simulink model "helicopter_control_xplane_9"  (R2016a)
settings: Solver=VariableStepAuto  StartTime=0.0  StopTime=inf  RelTol=1e-3
libraries: dspindex x18, dspnetwork x4, etargetslib x2
settings Model: Creator=iwin  LastModifiedBy=iwin

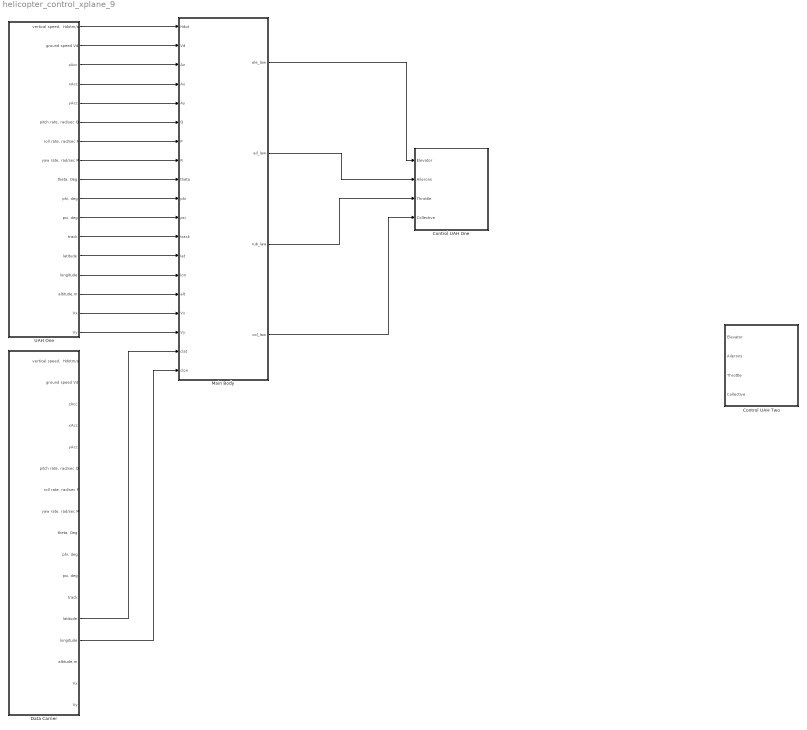
== system helicopter_control_xplane_9 ==
  Control UAH One : Subsystem  Description=|  mask(Send Commands to X-Plane 9){remoteURL='192.168.137.5', remotePort=49000}
      | Done by: Mohamed Abdelkader
      | Contact for updates: mohamedashraf123@gmail.com
      mask prompts: remoteURL "Remote X-Plane Address ('127.0.0.1')"; remotePort "Remote X-Plane Port (49000)"
      mask help:
      | Sends Control Surfaces Commands to Xplane 9
      | Throttle in [0,1]
      | Elevator, Ailerons, rudder, nosewheel in [-1,1]
      mask TypeOptions remoteURL: UDP Send/remoteURL
  Control UAH Two : Subsystem  Description=|  mask(Send Commands to X-Plane 9){remoteURL='192.168.137.6', remotePort=49000}
      | Done by: Mohamed Abdelkader
      | Contact for updates: mohamedashraf123@gmail.com
      mask prompts: remoteURL "Remote X-Plane Address ('127.0.0.1')"; remotePort "Remote X-Plane Port (49000)"
      mask help:
      | Sends Control Surfaces Commands to Xplane 9
      | Throttle in [0,1]
      | Elevator, Ailerons, rudder, nosewheel in [-1,1]
      mask TypeOptions remoteURL: UDP Send/remoteURL
  Data Carrier : Subsystem  Description=|  TreatAsAtomicUnit=on  mask(Get Data from Xplane10){remoteURL='192.168.137.6', localPort=49005, sampletime=0.02}
      | Done by: Mohamed Abdelkader
      | Contact for updates: mohamedashraf123@gmail.com
      mask prompts: remoteURL "Remote IP address ('0.0.0.0' to accept all):(default='127.0.0.1')"; localPort "Local IP port: that Xplane10 sends to (default=49005)"; sampletime "Sampling time (seconds), how frequenlty to capture data from Xplane. Don't set to low as it might not be able to capture the smaples from Xplane. Default is 0.02 assuming the UDP rate in Xplane is set to 50 sample per second"
      mask help:
      | Get Data from X-Plane10
      | * make sure you configure the right port
      | and the right IP address
      mask TypeOptions remoteURL: UDP Receive1/remoteURL
      mask TypeOptions localPort: UDP Receive1/localPort
      mask TypeOptions sampletime: UDP Receive1/sampletime
  Main Body : Subsystem  mask(Controller for Helicoper){PSICMD=0, VYCMD=0, VXCMD=0, HCMD=12}
      mask prompts: PSICMD "Give the yaw angle"; VYCMD "Give the latitude velocity"; VXCMD "Give the longitude velocity"; HCMD "Give the height"
      mask help: Control the Helicopter in X-Plane 9
  UAH One : Subsystem  Description=|  TreatAsAtomicUnit=on  mask(Get Data from Xplane10){remoteURL='192.168.137.5', localPort=49005, sampletime=0.02}
      | Done by: Mohamed Abdelkader
      | Contact for updates: mohamedashraf123@gmail.com
      mask prompts: remoteURL "Remote IP address ('0.0.0.0' to accept all):(default='127.0.0.1')"; localPort "Local IP port: that Xplane10 sends to (default=49005)"; sampletime "Sampling time (seconds), how frequenlty to capture data from Xplane. Don't set to low as it might not be able to capture the smaples from Xplane. Default is 0.02 assuming the UDP rate in Xplane is set to 50 sample per second"
      mask help:
      | Get Data from X-Plane10
      | * make sure you configure the right port
      | and the right IP address
      mask TypeOptions remoteURL: UDP Receive1/remoteURL
      mask TypeOptions localPort: UDP Receive1/localPort
      mask TypeOptions sampletime: UDP Receive1/sampletime
  wires:
  Main Body/1(ele_law) -> Control UAH One/1(Elevator)
  Main Body/2(ail_law) -> Control UAH One/2(Ailerons)
  Main Body/3(rub_law) -> Control UAH One/3(Throttle)
  Main Body/4(col_law) -> Control UAH One/4(Collective)
  UAH One/1("vertical speed,  Hdotm/s") -> Main Body/1(Hdot)
  UAH One/2(ground speed Vd) -> Main Body/2(Vd)
  UAH One/3(zAcc) -> Main Body/3(Az)
  UAH One/4(xAcc) -> Main Body/4(Ax)
  UAH One/5(yAcc) -> Main Body/5(Ay)
  UAH One/6("pitch rate, rad/sec Q") -> Main Body/6(Q)
  UAH One/7(" roll rate, rad/sec P") -> Main Body/7(P)
  UAH One/8("yaw rate, rad/sec R") -> Main Body/8(R)
  UAH One/9("theta, Deg") -> Main Body/9(theta)
  UAH One/10("phi, deg") -> Main Body/10(phi)
  UAH One/11("psi, deg") -> Main Body/11(psi)
  UAH One/12(track) -> Main Body/12(track)
  UAH One/13(latitude) -> Main Body/13(lat)
  UAH One/14(longitude) -> Main Body/14(lon)
  UAH One/15(altitude,m) -> Main Body/15(alt)
  UAH One/16(Vx) -> Main Body/16(Vx)
  UAH One/17(Vy) -> Main Body/17(Vy)
  Data Carrier/13(latitude) -> Main Body/18(clat)
  Data Carrier/14(longitude) -> Main Body/19(clon)

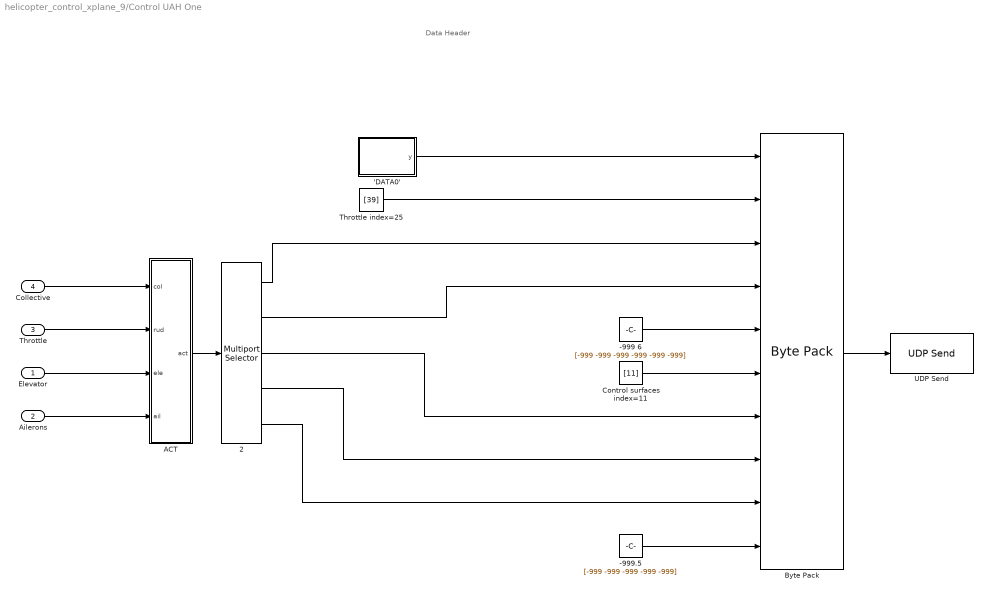
== system helicopter_control_xplane_9/Control UAH One ==
  note: Data Header
  Elevator : Inport
  Ailerons : Inport  Port=2
  Throttle : Inport  Port=3
  Collective : Inport  Port=4
  'DATA0' : MATLAB Function  TreatAsAtomicUnit=on
  -999 6 : Constant  Value=[-999 -999 -999 -999 -999 -999]  OutDataTypeStr=int32  SampleTime=-1
  -999.5 : Constant  Value=[-999 -999 -999 -999 -999]  OutDataTypeStr=int32  SampleTime=-1
  2 : dspindex/Multiport Selector  rowsOrCols=Columns  idxCellArray={1 2 3 4 5}  idxErrMode=Clip Index
  ACT : MATLAB Function  TreatAsAtomicUnit=on
  Byte Pack : etargetslib/Byte Pack  datatypes={'uint8','uint32','single','single','int32','uint32','single','single','single','int32'}  byteAlign=1
  Control surfaces index=11 : Constant  Value=[11]  OutDataTypeStr=uint32  SampleTime=-1
  Throttle index=25 : Constant  Value=[39]  OutDataTypeStr=uint32  SampleTime=-1
  UDP Send : dspnetwork/UDP Send  remoteURL=remoteURL  remotePort=49000  localURL='0.0.0.0'  localPortSource=Automatically determine  localPort=-1  sampletime=-1  separateLengthPort=0
  wires:
  Byte Pack/1 -> UDP Send/1
  Throttle index=25/1 -> Byte Pack/2
  'DATA0'/1(y) -> Byte Pack/1
  -999 6/1 -> Byte Pack/5
  Control surfaces index=11/1 -> Byte Pack/6
  -999.5/1 -> Byte Pack/10
  2/1 -> Byte Pack/3
  2/2 -> Byte Pack/4
  ACT/1(act) -> 2/1
  Collective/1 -> ACT/1(col)
  Elevator/1 -> ACT/3(ele)
  Throttle/1 -> ACT/2(rud)
  Ailerons/1 -> ACT/4(ail)
  2/3 -> Byte Pack/7
  2/4 -> Byte Pack/8
  2/5 -> Byte Pack/9

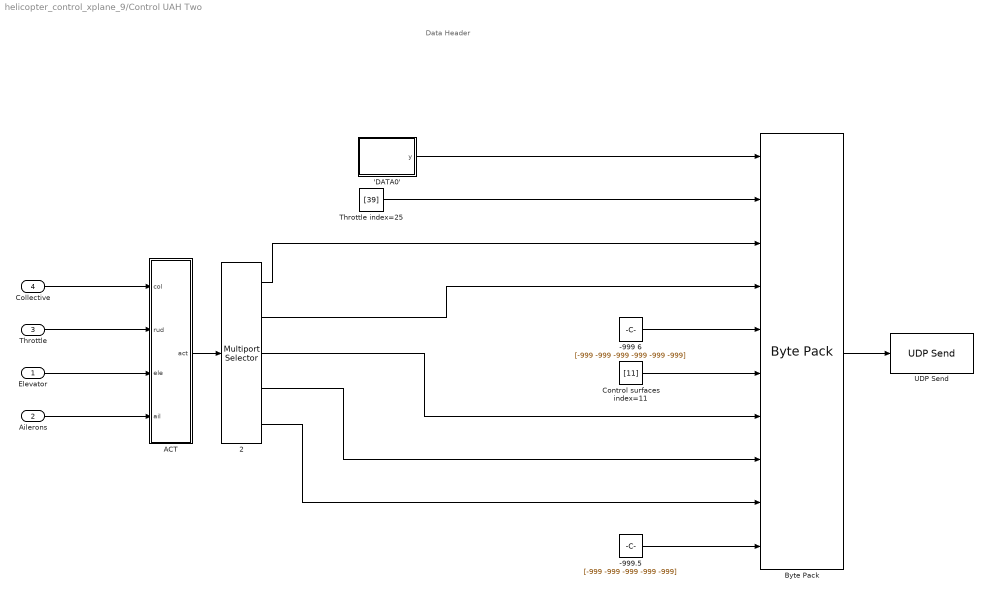
== system helicopter_control_xplane_9/Control UAH Two ==
  note: Data Header
  Elevator : Inport
  Ailerons : Inport  Port=2
  Throttle : Inport  Port=3
  Collective : Inport  Port=4
  'DATA0' : MATLAB Function  TreatAsAtomicUnit=on
  -999 6 : Constant  Value=[-999 -999 -999 -999 -999 -999]  OutDataTypeStr=int32  SampleTime=-1
  -999.5 : Constant  Value=[-999 -999 -999 -999 -999]  OutDataTypeStr=int32  SampleTime=-1
  2 : dspindex/Multiport Selector  rowsOrCols=Columns  idxCellArray={1 2 3 4 5}  idxErrMode=Clip Index
  ACT : MATLAB Function  TreatAsAtomicUnit=on
  Byte Pack : etargetslib/Byte Pack  datatypes={'uint8','uint32','single','single','int32','uint32','single','single','single','int32'}  byteAlign=1
  Control surfaces index=11 : Constant  Value=[11]  OutDataTypeStr=uint32  SampleTime=-1
  Throttle index=25 : Constant  Value=[39]  OutDataTypeStr=uint32  SampleTime=-1
  UDP Send : dspnetwork/UDP Send  remoteURL=remoteURL  remotePort=49000  localURL='0.0.0.0'  localPortSource=Automatically determine  localPort=-1  sampletime=-1  separateLengthPort=0
  wires:
  2/5 -> Byte Pack/9
  2/4 -> Byte Pack/8
  2/3 -> Byte Pack/7
  Ailerons/1 -> ACT/4(ail)
  Throttle/1 -> ACT/2(rud)
  Elevator/1 -> ACT/3(ele)
  Collective/1 -> ACT/1(col)
  ACT/1(act) -> 2/1
  2/2 -> Byte Pack/4
  2/1 -> Byte Pack/3
  -999.5/1 -> Byte Pack/10
  Control surfaces index=11/1 -> Byte Pack/6
  -999 6/1 -> Byte Pack/5
  'DATA0'/1(y) -> Byte Pack/1
  Throttle index=25/1 -> Byte Pack/2
  Byte Pack/1 -> UDP Send/1

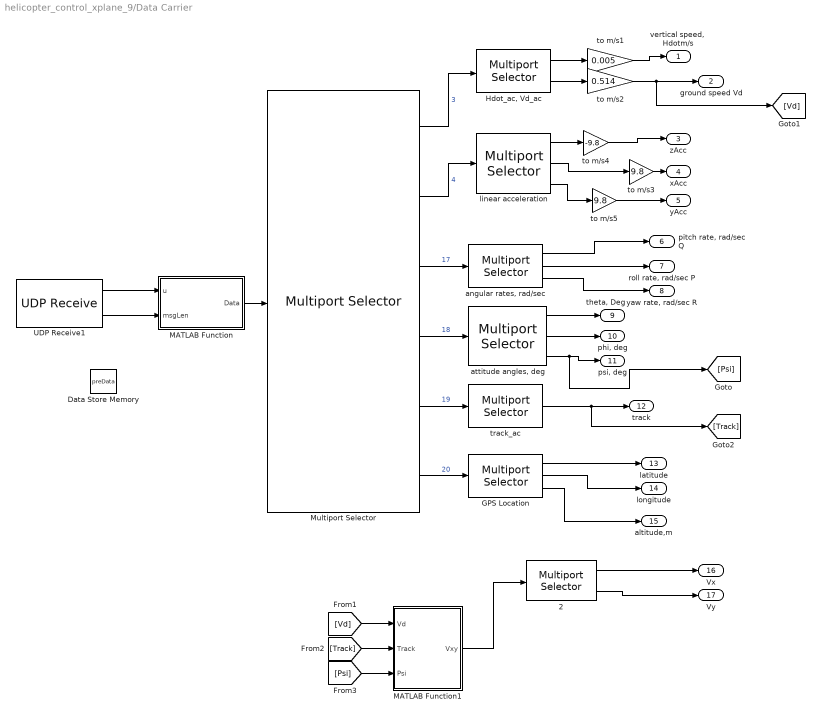
== system helicopter_control_xplane_9/Data Carrier ==
  2 : dspindex/Multiport Selector  rowsOrCols=Columns  idxCellArray={1 2}  idxErrMode=Clip Index
  Data Store Memory : DataStoreMemory  DataStoreName=preData  InitialValue=zeros(140, 8)  ShowAdditionalParam=off  OutDataTypeStr=single
  GPS Location : dspindex/Multiport Selector  rowsOrCols=Columns  idxCellArray={1,2,3}  idxErrMode=Clip Index
  "Hdot_ac, Vd_ac" : dspindex/Multiport Selector  rowsOrCols=Columns  idxCellArray={5, 7}  idxErrMode=Clip Index
  MATLAB Function : MATLAB Function  TreatAsAtomicUnit=on
  MATLAB Function1 : MATLAB Function  TreatAsAtomicUnit=on
  Multiport Selector : dspindex/Multiport Selector  rowsOrCols=Rows  idxCellArray={3,4,17,18,19,20}  idxErrMode=Clip Index
  UDP Receive1 : dspnetwork/UDP Receive  localURL='0.0.0.0'  localPort=localPort  remoteURL=remoteURL  remotePort=-1  recvBufferSize=8192  dims=365*20  signalDatatype=uint8  isVarSize=off  showBlockingTime=off  blockingTime=0  sampletime=sampletime
  "angular rates, rad/sec" : dspindex/Multiport Selector  rowsOrCols=Columns  idxCellArray={1,2,3}  idxErrMode=Clip Index
  "attitude angles, deg" : dspindex/Multiport Selector  rowsOrCols=Columns  idxCellArray={1, 2, 3}  idxErrMode=Clip Index
  linear acceleration : dspindex/Multiport Selector  rowsOrCols=Columns  idxCellArray={3, 4, 5}  idxErrMode=Clip Index
  to m/s1 : Gain  Gain=0.005  OutDataTypeStr=double
  to m/s2 : Gain  Gain=0.514
  to m/s3 : Gain  Gain=9.8
  to m/s4 : Gain  Gain=-9.8
  to m/s5 : Gain  Gain=9.8
  track_ac : dspindex/Multiport Selector  rowsOrCols=Columns  idxCellArray={3}  idxErrMode=Clip Index
  "vertical speed,  Hdotm/s" : Outport  OutDataTypeStr=double
  ground speed Vd : Outport  Port=2
  zAcc : Outport  Port=3
  xAcc : Outport  Port=4
  yAcc : Outport  Port=5
  "pitch rate, rad/sec Q" : Outport  Port=6
  " roll rate, rad/sec P" : Outport  Port=7
  "yaw rate, rad/sec R" : Outport  Port=8
  "theta, Deg" : Outport  Port=9
  "phi, deg" : Outport  Port=10
  "psi, deg" : Outport  Port=11
  track : Outport  Port=12
  latitude : Outport  Port=13
  longitude : Outport  Port=14
  altitude,m : Outport  Port=15
  Vx : Outport  Port=16
  Vy : Outport  Port=17
  wires:
  2/2 -> Vy/1
  2/1 -> Vx/1
  MATLAB Function1/1(Vxy) -> 2/1
  [Vd] -> MATLAB Function1/1(Vd)
  [Track] -> MATLAB Function1/2(Track)
  [Psi] -> MATLAB Function1/3(Psi)
  track_ac/1 -> track/1, [Track]
  "attitude angles, deg"/1 -> "theta, Deg"/1
  "angular rates, rad/sec"/1 -> "pitch rate, rad/sec Q"/1
  to m/s5/1 -> yAcc/1
  linear acceleration/3 -> to m/s5/1
  linear acceleration/2 -> to m/s3/1
  to m/s4/1 -> zAcc/1
  to m/s2/1 -> ground speed Vd/1, [Vd]
  to m/s1/1 -> "vertical speed,  Hdotm/s"/1
  "Hdot_ac, Vd_ac"/2 -> to m/s2/1
  "Hdot_ac, Vd_ac"/1 -> to m/s1/1
  Multiport Selector/6 -> GPS Location/1  "20"
  Multiport Selector/5 -> track_ac/1  "19"
  Multiport Selector/4 -> "attitude angles, deg"/1  "18"
  Multiport Selector/3 -> "angular rates, rad/sec"/1  "17"
  "attitude angles, deg"/2 -> "phi, deg"/1
  "attitude angles, deg"/3 -> "psi, deg"/1, [Psi]
  UDP Receive1/2 -> MATLAB Function/2(msgLen)
  UDP Receive1/1 -> MATLAB Function/1(u)
  GPS Location/3 -> altitude,m/1
  to m/s3/1 -> xAcc/1
  "angular rates, rad/sec"/2 -> " roll rate, rad/sec P"/1
  GPS Location/1 -> latitude/1
  linear acceleration/1 -> to m/s4/1
  GPS Location/2 -> longitude/1
  Multiport Selector/1 -> "Hdot_ac, Vd_ac"/1  "3"
  MATLAB Function/1(Data) -> Multiport Selector/1
  "angular rates, rad/sec"/3 -> "yaw rate, rad/sec R"/1
  Multiport Selector/2 -> linear acceleration/1  "4"

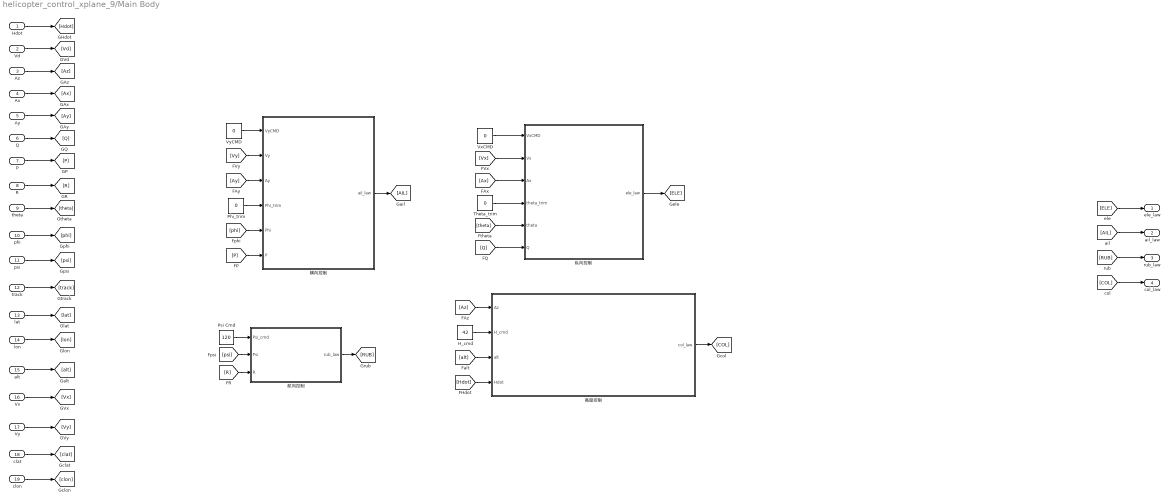
== system helicopter_control_xplane_9/Main Body ==
  Hdot : Inport
  Vd : Inport  Port=2
  Az : Inport  Port=3
  Ax : Inport  Port=4
  Ay : Inport  Port=5
  Q : Inport  Port=6
  P : Inport  Port=7
  R : Inport  Port=8
  theta : Inport  Port=9
  phi : Inport  Port=10
  psi : Inport  Port=11
  track : Inport  Port=12
  lat : Inport  Port=13
  lon : Inport  Port=14
  alt : Inport  Port=15
  Vx : Inport  Port=16
  Vy : Inport  Port=17
  clat : Inport  Port=18
  clon : Inport  Port=19
  H_cmd : Constant  Value=42  OutDataTypeStr=single
  Phi_trim : Constant  Value=0  OutDataTypeStr=single
  Psi Cmd : Constant  Value=120  OutDataTypeStr=single
  Theta_trim : Constant  Value=0  OutDataTypeStr=single
  VxCMD : Constant  Value=0  OutDataTypeStr=single
  VyCMD : Constant  Value=0  OutDataTypeStr=single
  横向控制 : Subsystem
  纵向控制 : Subsystem
  航向控制 : Subsystem
  高度控制 : Subsystem
  ele_law : Outport
  ail_law : Outport  Port=2
  rub_law : Outport  Port=3
  col_law : Outport  Port=4
  wires:
  Hdot/1 -> [Hdot]
  Vd/1 -> [Vd]
  Az/1 -> [Az]
  Ax/1 -> [Ax]
  Ay/1 -> [Ay]
  Q/1 -> [Q]
  P/1 -> [P]
  R/1 -> [R]
  theta/1 -> [theta]
  phi/1 -> [phi]
  psi/1 -> [psi]
  track/1 -> [track]
  lat/1 -> [lat]
  lon/1 -> [lon]
  alt/1 -> [alt]
  [ELE] -> ele_law/1
  [AIL] -> ail_law/1
  [RUB] -> rub_law/1
  [COL] -> col_law/1
  Vx/1 -> [Vx]
  Vy/1 -> [Vy]
  [Az] -> 高度控制/1(Az)
  H_cmd/1 -> 高度控制/2(H_cmd)
  [alt] -> 高度控制/3(alt)
  [Hdot] -> 高度控制/4(Hdot)
  高度控制/1(col_law) -> [COL]
  Psi Cmd/1 -> 航向控制/1(Psi_cmd)
  [psi] -> 航向控制/2(Psi)
  [R] -> 航向控制/3(R)
  航向控制/1(rub_law) -> [RUB]
  VyCMD/1 -> 横向控制/1(VyCMD)
  [Vy] -> 横向控制/2(Vy)
  [Ay] -> 横向控制/3(Ay)
  Phi_trim/1 -> 横向控制/4(Phi_trim)
  [phi] -> 横向控制/5(Phi)
  [P] -> 横向控制/6(P)
  横向控制/1(ail_law) -> [AIL]
  VxCMD/1 -> 纵向控制/1(VxCMD)
  [Vx] -> 纵向控制/2(Vx)
  [Ax] -> 纵向控制/3(Ax)
  Theta_trim/1 -> 纵向控制/4(theta_trim)
  [theta] -> 纵向控制/5(theta)
  [Q] -> 纵向控制/6(Q)
  纵向控制/1(ele_law) -> [ELE]
  clat/1 -> [clat]
  clon/1 -> [clon]

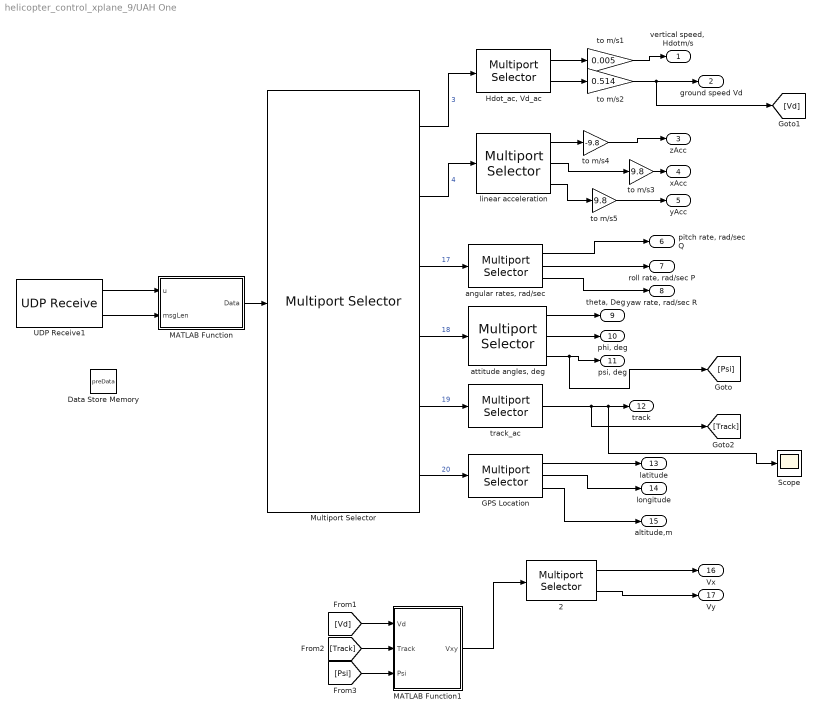
== system helicopter_control_xplane_9/UAH One ==
  2 : dspindex/Multiport Selector  rowsOrCols=Columns  idxCellArray={1 2}  idxErrMode=Clip Index
  Data Store Memory : DataStoreMemory  DataStoreName=preData  InitialValue=zeros(140, 8)  ShowAdditionalParam=off  OutDataTypeStr=single
  GPS Location : dspindex/Multiport Selector  rowsOrCols=Columns  idxCellArray={1,2,3}  idxErrMode=Clip Index
  "Hdot_ac, Vd_ac" : dspindex/Multiport Selector  rowsOrCols=Columns  idxCellArray={5, 7}  idxErrMode=Clip Index
  MATLAB Function : MATLAB Function  TreatAsAtomicUnit=on
  MATLAB Function1 : MATLAB Function  TreatAsAtomicUnit=on
  Multiport Selector : dspindex/Multiport Selector  rowsOrCols=Rows  idxCellArray={3,4,17,18,19,20}  idxErrMode=Clip Index
  Scope : Scope
  UDP Receive1 : dspnetwork/UDP Receive  localURL='0.0.0.0'  localPort=localPort  remoteURL=remoteURL  remotePort=-1  recvBufferSize=8192  dims=365*20  signalDatatype=uint8  isVarSize=off  showBlockingTime=off  blockingTime=0  sampletime=sampletime
  "angular rates, rad/sec" : dspindex/Multiport Selector  rowsOrCols=Columns  idxCellArray={1,2,3}  idxErrMode=Clip Index
  "attitude angles, deg" : dspindex/Multiport Selector  rowsOrCols=Columns  idxCellArray={1, 2, 3}  idxErrMode=Clip Index
  linear acceleration : dspindex/Multiport Selector  rowsOrCols=Columns  idxCellArray={3, 4, 5}  idxErrMode=Clip Index
  to m/s1 : Gain  Gain=0.005  OutDataTypeStr=double
  to m/s2 : Gain  Gain=0.514
  to m/s3 : Gain  Gain=9.8
  to m/s4 : Gain  Gain=-9.8
  to m/s5 : Gain  Gain=9.8
  track_ac : dspindex/Multiport Selector  rowsOrCols=Columns  idxCellArray={3}  idxErrMode=Clip Index
  "vertical speed,  Hdotm/s" : Outport  OutDataTypeStr=double
  ground speed Vd : Outport  Port=2
  zAcc : Outport  Port=3
  xAcc : Outport  Port=4
  yAcc : Outport  Port=5
  "pitch rate, rad/sec Q" : Outport  Port=6
  " roll rate, rad/sec P" : Outport  Port=7
  "yaw rate, rad/sec R" : Outport  Port=8
  "theta, Deg" : Outport  Port=9
  "phi, deg" : Outport  Port=10
  "psi, deg" : Outport  Port=11
  track : Outport  Port=12
  latitude : Outport  Port=13
  longitude : Outport  Port=14
  altitude,m : Outport  Port=15
  Vx : Outport  Port=16
  Vy : Outport  Port=17
  wires:
  Multiport Selector/2 -> linear acceleration/1  "4"
  "angular rates, rad/sec"/3 -> "yaw rate, rad/sec R"/1
  MATLAB Function/1(Data) -> Multiport Selector/1
  Multiport Selector/1 -> "Hdot_ac, Vd_ac"/1  "3"
  GPS Location/2 -> longitude/1
  linear acceleration/1 -> to m/s4/1
  GPS Location/1 -> latitude/1
  "angular rates, rad/sec"/2 -> " roll rate, rad/sec P"/1
  to m/s3/1 -> xAcc/1
  GPS Location/3 -> altitude,m/1
  UDP Receive1/1 -> MATLAB Function/1(u)
  UDP Receive1/2 -> MATLAB Function/2(msgLen)
  "attitude angles, deg"/3 -> [Psi], "psi, deg"/1
  "attitude angles, deg"/2 -> "phi, deg"/1
  Multiport Selector/3 -> "angular rates, rad/sec"/1  "17"
  Multiport Selector/4 -> "attitude angles, deg"/1  "18"
  Multiport Selector/5 -> track_ac/1  "19"
  Multiport Selector/6 -> GPS Location/1  "20"
  "Hdot_ac, Vd_ac"/1 -> to m/s1/1
  "Hdot_ac, Vd_ac"/2 -> to m/s2/1
  to m/s1/1 -> "vertical speed,  Hdotm/s"/1
  to m/s2/1 -> [Vd], ground speed Vd/1
  to m/s4/1 -> zAcc/1
  linear acceleration/2 -> to m/s3/1
  linear acceleration/3 -> to m/s5/1
  to m/s5/1 -> yAcc/1
  "angular rates, rad/sec"/1 -> "pitch rate, rad/sec Q"/1
  "attitude angles, deg"/1 -> "theta, Deg"/1
  track_ac/1 -> [Track], Scope/1, track/1
  [Psi] -> MATLAB Function1/3(Psi)
  [Track] -> MATLAB Function1/2(Track)
  [Vd] -> MATLAB Function1/1(Vd)
  MATLAB Function1/1(Vxy) -> 2/1
  2/1 -> Vx/1
  2/2 -> Vy/1

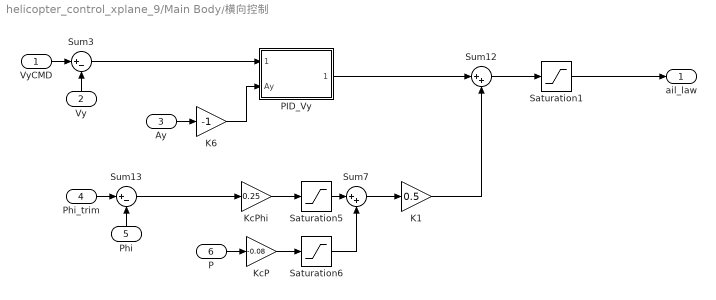
== system helicopter_control_xplane_9/Main Body/横向控制 ==
  VyCMD : Inport
  Vy : Inport  Port=2
  Ay : Inport  Port=3
  Phi_trim : Inport  Port=4
  Phi : Inport  Port=5
  P : Inport  Port=6
  K1 : Gain  Gain=0.5  OutDataTypeStr=single
  K6 : Gain  Gain=-1
  KcP : Gain  Gain=-0.08
  KcPhi : Gain  Gain=0.25  OutDataTypeStr=single
  PID_Vy : Subsystem
  Saturation1 : Saturate  UpperLimit=5.0  LowerLimit=-5.0
  Saturation5 : Saturate  UpperLimit=30  LowerLimit=-30
  Saturation6 : Saturate  UpperLimit=50  LowerLimit=-50
  Sum12 : Sum  Inputs=|++  AccumDataTypeStr=single  OutDataTypeStr=single  InputSameDT=on
  Sum13 : Sum  Inputs=|+-  OutDataTypeStr=double  InputSameDT=on
  Sum3 : Sum  Inputs=|+-  OutDataTypeStr=double  InputSameDT=on
  Sum7 : Sum  Inputs=|++  AccumDataTypeStr=single  OutDataTypeStr=double  InputSameDT=on
  ail_law : Outport
  wires:
  K6/1 -> PID_Vy/2(Ay)
  KcPhi/1 -> Saturation5/1
  Sum13/1 -> KcPhi/1
  KcP/1 -> Saturation6/1
  PID_Vy/1(AIL_FFC) -> Sum12/1
  Sum7/1 -> K1/1
  Saturation6/1 -> Sum7/2
  Saturation5/1 -> Sum7/1
  Sum3/1 -> PID_Vy/1(Vy_delta)
  Sum12/1 -> Saturation1/1
  K1/1 -> Sum12/2
  Phi/1 -> Sum13/2
  Ay/1 -> K6/1
  P/1 -> KcP/1
  Vy/1 -> Sum3/2
  Phi_trim/1 -> Sum13/1
  Saturation1/1 -> ail_law/1
  VyCMD/1 -> Sum3/1

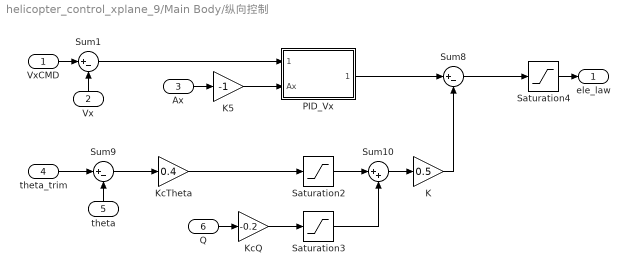
== system helicopter_control_xplane_9/Main Body/纵向控制 ==
  VxCMD : Inport
  Vx : Inport  Port=2
  Ax : Inport  Port=3
  theta_trim : Inport  Port=4
  theta : Inport  Port=5
  Q : Inport  Port=6
  K : Gain  Gain=0.5  OutDataTypeStr=single
  K5 : Gain  Gain=-1
  KcQ : Gain  Gain=-0.2
  KcTheta : Gain  Gain=0.4  OutDataTypeStr=single
  PID_Vx : Subsystem
  Saturation2 : Saturate  UpperLimit=45  LowerLimit=-45
  Saturation3 : Saturate  UpperLimit=50  LowerLimit=-50
  Saturation4 : Saturate  UpperLimit=5.0  LowerLimit=-5.0
  Sum1 : Sum  Inputs=|+-  OutDataTypeStr=double  InputSameDT=on
  Sum10 : Sum  Inputs=|++  AccumDataTypeStr=single  OutDataTypeStr=double  InputSameDT=on
  Sum8 : Sum  Inputs=|+-  AccumDataTypeStr=single  OutMin=[-1]  OutMax=[1]  OutDataTypeStr=single  InputSameDT=on
  Sum9 : Sum  Inputs=|+-  OutDataTypeStr=double  InputSameDT=on
  ele_law : Outport
  wires:
  K5/1 -> PID_Vx/2(Ax)
  Sum10/1 -> K/1
  Sum8/1 -> Saturation4/1
  PID_Vx/1(ELE_FFC) -> Sum8/1
  KcQ/1 -> Saturation3/1
  Sum1/1 -> PID_Vx/1(Vx_delta)
  Saturation2/1 -> Sum10/1
  K/1 -> Sum8/2
  KcTheta/1 -> Saturation2/1
  Saturation3/1 -> Sum10/2
  Sum9/1 -> KcTheta/1
  Vx/1 -> Sum1/2
  VxCMD/1 -> Sum1/1
  Saturation4/1 -> ele_law/1
  Ax/1 -> K5/1
  theta_trim/1 -> Sum9/1
  theta/1 -> Sum9/2
  Q/1 -> KcQ/1

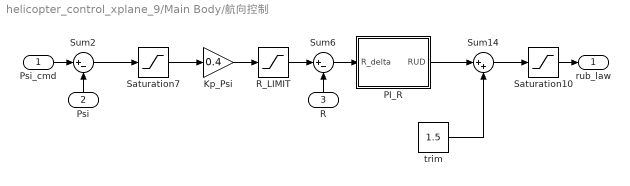
== system helicopter_control_xplane_9/Main Body/航向控制 ==
  Psi_cmd : Inport
  Psi : Inport  Port=2
  R : Inport  Port=3
  Kp_Psi : Gain  Gain=0.4  OutDataTypeStr=single
  PI_R : Subsystem
  R_LIMIT : Saturate  UpperLimit=5  LowerLimit=-5
  Saturation10 : Saturate  UpperLimit=20.0  LowerLimit=-8.0  OutDataTypeStr=single
  Saturation7 : Saturate  UpperLimit=30  LowerLimit=-30
  Sum14 : Sum  Inputs=|++  OutMin=[-1]  OutMax=[1]  OutDataTypeStr=double  InputSameDT=on
  Sum2 : Sum  Inputs=|+-  OutDataTypeStr=double  InputSameDT=on
  Sum6 : Sum  Inputs=|+-  OutDataTypeStr=double  InputSameDT=on
  trim : Constant  Value=1.5  OutDataTypeStr=single
  rub_law : Outport
  wires:
  R_LIMIT/1 -> Sum6/1
  Sum2/1 -> Saturation7/1
  trim/1 -> Sum14/2
  Kp_Psi/1 -> R_LIMIT/1
  Saturation7/1 -> Kp_Psi/1
  PI_R/1(RUD) -> Sum14/1
  Sum6/1 -> PI_R/1(R_delta)
  Sum14/1 -> Saturation10/1
  Saturation10/1 -> rub_law/1
  Psi_cmd/1 -> Sum2/1
  Psi/1 -> Sum2/2
  R/1 -> Sum6/2

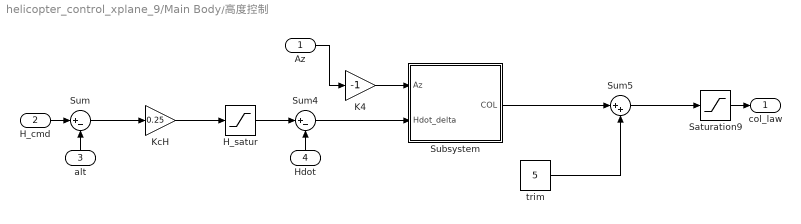
== system helicopter_control_xplane_9/Main Body/高度控制 ==
  Az : Inport
  H_cmd : Inport  Port=2
  alt : Inport  Port=3
  Hdot : Inport  Port=4
  H_satur : Saturate  UpperLimit=1.0  LowerLimit=-1.0
  K4 : Gain  Gain=-1
  KcH : Gain  Gain=0.25
  Saturation9 : Saturate  UpperLimit=10  LowerLimit=0
  Subsystem : Subsystem
  Sum : Sum  Inputs=|+-  OutDataTypeStr=double  InputSameDT=on
  Sum4 : Sum  Inputs=|+-  OutDataTypeStr=single  InputSameDT=on
  Sum5 : Sum  Inputs=|++  OutMin=[-1]  OutMax=[1]  OutDataTypeStr=double  InputSameDT=on
  trim : Constant  Value=5  OutDataTypeStr=single
  col_law : Outport
  wires:
  Sum/1 -> KcH/1
  KcH/1 -> H_satur/1
  H_satur/1 -> Sum4/1
  Subsystem/1(COL) -> Sum5/1
  trim/1 -> Sum5/2
  Sum5/1 -> Saturation9/1
  Sum4/1 -> Subsystem/2(Hdot_delta)
  K4/1 -> Subsystem/1(Az)
  H_cmd/1 -> Sum/1
  alt/1 -> Sum/2
  Az/1 -> K4/1
  Hdot/1 -> Sum4/2
  Saturation9/1 -> col_law/1

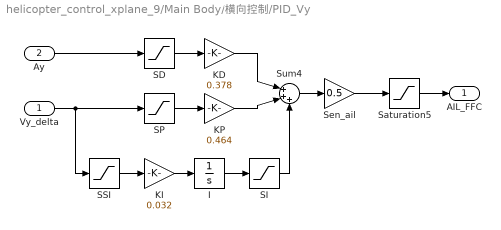
== system helicopter_control_xplane_9/Main Body/横向控制/PID_Vy ==
  Vy_delta : Inport
  Ay : Inport  Port=2
  I : Integrator
  KD : Gain  Gain=0.378  OutDataTypeStr=single
  KI : Gain  Gain=0.032
  KP : Gain  Gain=0.464  OutDataTypeStr=single
  SD : Saturate  UpperLimit=2.0  LowerLimit=-2.0
  SI : Saturate  UpperLimit=3.0  LowerLimit=-3.0  OutDataTypeStr=single
  SP : Saturate  UpperLimit=4.0  LowerLimit=-4.0
  SSI : Saturate  UpperLimit=2.0  LowerLimit=-2.0
  Saturation5 : Saturate  UpperLimit=5.0  LowerLimit=-5.0  OutDataTypeStr=single
  Sen_ail : Gain  Gain=0.5
  Sum4 : Sum  Inputs=|+++  AccumDataTypeStr=single  OutMin=[-20]  OutMax=[20]  OutDataTypeStr=double  InputSameDT=on
  AIL_FFC : Outport  OutDataTypeStr=single
  wires:
  Sen_ail/1 -> Saturation5/1
  KD/1 -> Sum4/1
  SD/1 -> KD/1
  Ay/1 -> SD/1
  KP/1 -> Sum4/2
  SI/1 -> Sum4/3
  Saturation5/1 -> AIL_FFC/1
  Sum4/1 -> Sen_ail/1
  KI/1 -> I/1
  I/1 -> SI/1
  Vy_delta/1 -> SP/1, SSI/1
  SP/1 -> KP/1
  SSI/1 -> KI/1

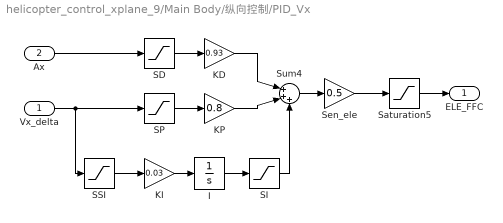
== system helicopter_control_xplane_9/Main Body/纵向控制/PID_Vx ==
  Vx_delta : Inport
  Ax : Inport  Port=2
  I : Integrator
  KD : Gain  Gain=0.93  OutDataTypeStr=single
  KI : Gain  Gain=0.03  ParamDataTypeStr=single  OutDataTypeStr=double
  KP : Gain  Gain=0.8  OutDataTypeStr=single
  SD : Saturate  UpperLimit=5.0  LowerLimit=-5.0
  SI : Saturate  UpperLimit=3.0  LowerLimit=-3.0  OutDataTypeStr=single
  SP : Saturate  UpperLimit=4.0  LowerLimit=-4.0
  SSI : Saturate  UpperLimit=2.0  LowerLimit=-2.0  OutDataTypeStr=single
  Saturation5 : Saturate  UpperLimit=5.0  LowerLimit=-5.0  OutDataTypeStr=single
  Sen_ele : Gain  Gain=0.5  OutDataTypeStr=single
  Sum4 : Sum  Inputs=|+++  AccumDataTypeStr=single  OutMin=[-20]  OutMax=[20]  OutDataTypeStr=single  InputSameDT=on
  ELE_FFC : Outport  OutDataTypeStr=single
  wires:
  SI/1 -> Sum4/3
  KD/1 -> Sum4/1
  Ax/1 -> SD/1
  SSI/1 -> KI/1
  SP/1 -> KP/1
  Vx_delta/1 -> SSI/1, SP/1
  I/1 -> SI/1
  KI/1 -> I/1
  Sum4/1 -> Sen_ele/1
  Saturation5/1 -> ELE_FFC/1
  KP/1 -> Sum4/2
  SD/1 -> KD/1
  Sen_ele/1 -> Saturation5/1

== system helicopter_control_xplane_9/Main Body/航向控制/PI_R ==
  R_delta : Inport
  I : Integrator
  Ki_R : Gain  Gain=0.05
  Kp_R : Gain  Gain=0.5
  SI : Saturate  UpperLimit=10.0  LowerLimit=-8.0
  SP : Saturate  UpperLimit=30  LowerLimit=-30
  SSI : Saturate  UpperLimit=10  LowerLimit=-10
  Sen_rud : Gain  Gain=0.5  OutDataTypeStr=single
  Sum4 : Sum  Inputs=|++  OutMin=[-20]  OutMax=[20]  OutDataTypeStr=double  InputSameDT=on
  RUD : Outport  OutDataTypeStr=single
  wires:
  SI/1 -> Sum4/2
  Kp_R/1 -> Sum4/1
  SSI/1 -> Ki_R/1
  SP/1 -> Kp_R/1
  R_delta/1 -> SSI/1, SP/1
  I/1 -> SI/1
  Ki_R/1 -> I/1
  Sum4/1 -> Sen_rud/1
  Sen_rud/1 -> RUD/1

== system helicopter_control_xplane_9/Main Body/高度控制/Subsystem ==
  Az : Inport
  Hdot_delta : Inport  Port=2
  I : Integrator
  KcP1 : Gain  Gain=0.5  OutDataTypeStr=single
  Ki_Hdot : Gain  Gain=0.05  OutDataTypeStr=double
  Kp_Hdot : Gain  Gain=0.5  OutDataTypeStr=single
  SD : Saturate  UpperLimit=3.0  LowerLimit=-3.0
  SI : Saturate  UpperLimit=2.0  LowerLimit=-2.0  OutDataTypeStr=single
  SP : Saturate  UpperLimit=4.0  LowerLimit=-4.0
  SSI : Saturate  UpperLimit=1.0  LowerLimit=-1.0
  Sen_col : Gain  Gain=0.5  OutDataTypeStr=single
  Sum5 : Sum  Inputs=|+++  AccumDataTypeStr=single  OutMin=[-20]  OutMax=[20]  OutDataTypeStr=single  InputSameDT=on
  COL : Outport  OutDataTypeStr=single
  wires:
  Az/1 -> SD/1
  SD/1 -> KcP1/1
  KcP1/1 -> Sum5/1
  Hdot_delta/1 -> SSI/1, SP/1
  SSI/1 -> Ki_Hdot/1
  Ki_Hdot/1 -> I/1
  SP/1 -> Kp_Hdot/1
  Kp_Hdot/1 -> Sum5/2
  I/1 -> SI/1
  SI/1 -> Sum5/3
  Sen_col/1 -> COL/1
  Sum5/1 -> Sen_col/1

== matlab function helicopter_control_xplane_9/UAH One/MATLAB Function ==
  data: u input uint8; Data output single size=[140 8]; msgLen input; preData data_store_memory
% 
% Handle the data received from x-plane 9
% 
% Author: Gui Zhou
% Date: 2017-02-14
%

function Data  = fcn(u,msgLen)
    %#codegen
    global preData; 
    %coder.extrinsic('clear')
    dataLen=msgLen-5;
    Npackets=dataLen/36; 
    % initialize data matrix
    % rows: packets of data; columns: data values, first column is the data
    % index  



    maxNPackets=140;
    Nvalues=8;% number of values in each packet
    Data=single(zeros(maxNPackets,Nvalues));

    if dataLen > 0 

        Bytecounter=6; % start after the 5th byte 
        for j=1:Npackets
                        indx=typecast(u(Bytecounter:Bytecounter+3),'uint32');% packet index
                        %Data(indx,1)=single(indx); % packet index
                        Bytecounter=Bytecounter+4; % go to the next 4 bytes
                        Data(indx,1)=typecast(u(Bytecounter:Bytecounter+3),'single'); % 1st value
                        Bytecounter=Bytecounter+4; % go to the next 4 bytes
                        Data(indx,2)=typecast(u(Bytecounter:Bytecounter+3),'single'); % 2nd value
                        Bytecounter=Bytecounter+4; % go to the next 4 bytes
                        Data(indx,3)=typecast(u(Bytecounter:Bytecounter+3),'single'); % 3rd value
                        Bytecounter=Bytecounter+4; % go to the next 4 bytes
                        Data(indx,4)=typecast(u(Bytecounter:Bytecounter+3),'single'); % 4th value
                        Bytecounter=Bytecounter+4; % go to the next 4 bytes
                        Data(indx,5)=typecast(u(Bytecounter:Bytecounter+3),'single'); % 5th value
                        Bytecounter=Bytecounter+4; % go to the next 4 bytes
                        Data(indx,6)=typecast(u(Bytecounter:Bytecounter+3),'single'); % 6th value
                        Bytecounter=Bytecounter+4; % go to the next 4 bytes
                        Data(indx,7)=typecast(u(Bytecounter:Bytecounter+3),'single'); % 7th value
                        Bytecounter=Bytecounter+4; % go to the next 4 bytes
                        Data(indx,8)=typecast(u(Bytecounter:Bytecounter+3),'single'); % 8th value
                        Bytecounter=Bytecounter+4;% go to the next packet index 
        end  
        
        preData = Data;

    else 

        Data = preData;
   
    end
end



%clear Data

== matlab function helicopter_control_xplane_9/Control UAH One/'DATA0' ==
  data: y output
function y = fcn()
%#codegen
%y=uint8(zeros(1,77));
y = uint8('DATA0');

== matlab function helicopter_control_xplane_9/UAH One/MATLAB Function1 ==
  data: Vd input; Vxy output size=[1 2]; Track input; Psi input
function Vxy  = fcn(Vd,Track,Psi)
    Vxy=single(zeros(1,2));
	Vxy(1,1)=Vd*cos((Track-Psi)/57.3);
	Vxy(1,2)=Vd*sin((Track-Psi)/57.3);
end
%clear Data

== matlab function helicopter_control_xplane_9/Control UAH One/ACT ==
  data: act output size=[1 5]; col input; rud input; ele input; ail input
function act  = fcn(col,rud,ele,ail)
    act=single(zeros(1,5));
	act(1,1)=col;
    act(1,2)=-(rud-5.0)*2.0;
	act(1,5)=(rud-5.0)/10.0;
    act(1,3)=-(ele/5.0);
    act(1,4)=ail/5.0;
end

== matlab function helicopter_control_xplane_9/Data Carrier/MATLAB Function ==
  data: u input uint8; Data output single size=[140 8]; msgLen input; preData data_store_memory
% 
% Handle the data received from x-plane 9
% 
% Author: Gui Zhou
% Date: 2017-02-14
%

function Data  = fcn(u,msgLen)
    %#codegen
    global preData; 
    %coder.extrinsic('clear')
    dataLen=msgLen-5;
    Npackets=dataLen/36; 
    % initialize data matrix
    % rows: packets of data; columns: data values, first column is the data
    % index  



    maxNPackets=140;
    Nvalues=8;% number of values in each packet
    Data=single(zeros(maxNPackets,Nvalues));

    if dataLen > 0 

        Bytecounter=6; % start after the 5th byte 
        for j=1:Npackets
                        indx=typecast(u(Bytecounter:Bytecounter+3),'uint32');% packet index
                        %Data(indx,1)=single(indx); % packet index
                        Bytecounter=Bytecounter+4; % go to the next 4 bytes
                        Data(indx,1)=typecast(u(Bytecounter:Bytecounter+3),'single'); % 1st value
                        Bytecounter=Bytecounter+4; % go to the next 4 bytes
                        Data(indx,2)=typecast(u(Bytecounter:Bytecounter+3),'single'); % 2nd value
                        Bytecounter=Bytecounter+4; % go to the next 4 bytes
                        Data(indx,3)=typecast(u(Bytecounter:Bytecounter+3),'single'); % 3rd value
                        Bytecounter=Bytecounter+4; % go to the next 4 bytes
                        Data(indx,4)=typecast(u(Bytecounter:Bytecounter+3),'single'); % 4th value
                        Bytecounter=Bytecounter+4; % go to the next 4 bytes
                        Data(indx,5)=typecast(u(Bytecounter:Bytecounter+3),'single'); % 5th value
                        Bytecounter=Bytecounter+4; % go to the next 4 bytes
                        Data(indx,6)=typecast(u(Bytecounter:Bytecounter+3),'single'); % 6th value
                        Bytecounter=Bytecounter+4; % go to the next 4 bytes
                        Data(indx,7)=typecast(u(Bytecounter:Bytecounter+3),'single'); % 7th value
                        Bytecounter=Bytecounter+4; % go to the next 4 bytes
                        Data(indx,8)=typecast(u(Bytecounter:Bytecounter+3),'single'); % 8th value
                        Bytecounter=Bytecounter+4;% go to the next packet index 
        end  
        
        preData = Data;

    else 

        Data = preData;
   
    end
end



%clear Data

== matlab function helicopter_control_xplane_9/Data Carrier/MATLAB Function1 ==
  data: Vd input; Vxy output size=[1 2]; Track input; Psi input
function Vxy  = fcn(Vd,Track,Psi)
    Vxy=single(zeros(1,2));
	Vxy(1,1)=Vd*cos((Track-Psi)/57.3);
	Vxy(1,2)=Vd*sin((Track-Psi)/57.3);
end
%clear Data

== matlab function helicopter_control_xplane_9/Control UAH Two/'DATA0' ==
  data: y output
function y = fcn()
%#codegen
%y=uint8(zeros(1,77));
y = uint8('DATA0');

== matlab function helicopter_control_xplane_9/Control UAH Two/ACT ==
  data: act output size=[1 5]; col input; rud input; ele input; ail input
function act  = fcn(col,rud,ele,ail)
    act=single(zeros(1,5));
	act(1,1)=col;
    act(1,2)=-(rud-5.0)*2.0;
	act(1,5)=(rud-5.0)/10.0;
    act(1,3)=-(ele/5.0);
    act(1,4)=ail/5.0;
end
